simulink model "ms_inter5"  (Simulink 7.3)
settings: Solver=VariableStepDiscrete  StartTime=0.0  StopTime=10.0  MaxStep=0.1  RelTol=1e-3
undefined symbols (not defined in the file or in its folder): alge_calc
settings Model: Creator=sn00632  LastModifiedBy=sn00632

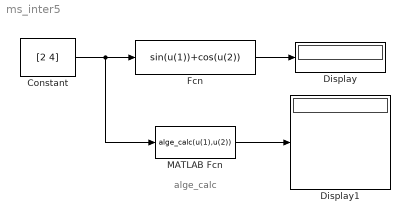
== system ms_inter5 ==
  note: alge_calc
  Constant : Constant  Value=[2 4]  OutDataType=fixdt(1, 16)  OutScaling=2^0
  Display : Display
  Display1 : Display
  Fcn : Fcn  Expr=sin(u(1))+cos(u(2))
  MATLAB Fcn : MATLABFcn  MATLABFcn=alge_calc(u(1),u(2))  OutputDimensions=5
  wires:
  Constant/1 -> Fcn/1, MATLAB Fcn/1
  Fcn/1 -> Display/1
  MATLAB Fcn/1 -> Display1/1
